simulink model "massMatrixTest"  (Simulink 7.9)
settings: Solver=FixedStepDiscrete  StartTime=0.0  StopTime=3  FixedStep=1  RelTol=1e-3
undefined symbols (not defined in the file or in its folder): robotName
libraries: utility x1
settings Model: Creator=jorhabib  LastModifiedBy=jorhabib

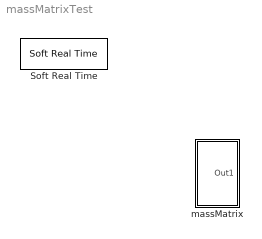
== system massMatrixTest ==
  Soft Real Time : utility/Soft Real Time  x=1
  massMatrix : Subsystem  mask{val=8, robotname=robotName, localname='simulink'}
      mask prompts: val "Block type"; robotname "Robot name"; localname "Module name"

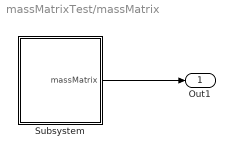
== system massMatrixTest/massMatrix ==
  Subsystem : Subsystem
  Out1 : Outport
  wires:
  Subsystem/1(massMatrix) -> Out1/1

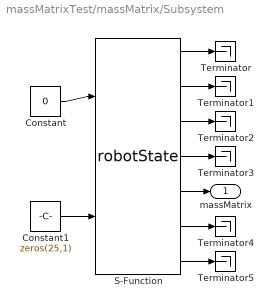
== system massMatrixTest/massMatrix/Subsystem ==
  Constant : Constant  Value=0  OutDataTypeStr=int8  SampleTime=-1
  Constant1 : Constant  Value=zeros(25,1)  OutDataTypeStr=double  SampleTime=-1
  S-Function : S-Function  FunctionName=robotState  Parameters=val,robotname,localname  EnableBusSupport=off
  Terminator{,1..5} (6 alike) : Terminator
  massMatrix : Outport
  wires:
  Constant/1 -> S-Function/1
  Constant1/1 -> S-Function/2
  S-Function/5 -> massMatrix/1
  S-Function/1 -> Terminator/1
  S-Function/2 -> Terminator1/1
  S-Function/3 -> Terminator2/1
  S-Function/4 -> Terminator3/1
  S-Function/6 -> Terminator4/1
  S-Function/7 -> Terminator5/1
